simulink model "model_dyskretny"  (R2023a)
settings: Solver=VariableStepAuto  StartTime=0.0  StopTime=200  RelTol=1e-3
values from neighbouring files (symbols this model uses):
  a0 = 0.000531632    [zad1.m]    (also in zad2_8.m; zadanie_dodatkowe.m)
  a1 = 0.0207337    [zad1.m]    (also in zad2_8.m; zadanie_dodatkowe.m)
  a2 = 0.254652    [zad1.m]    (also in zad2_8.m; zadanie_dodatkowe.m)
  alpha1 = -0.3    [zad1.m]    (also in zad2_8.m; zadanie_dodatkowe.m)
  alpha2 = -0.55    [zad1.m]    (also in zad2_8.m; zadanie_dodatkowe.m)
  alpha3 = 0.4    [zad1.m]    (also in zad2_8.m; zadanie_dodatkowe.m)
  alpha4 = 0.21    [zad1.m]    (also in zad2_8.m; zadanie_dodatkowe.m)
  b0 = 0.00122807    [zad1.m]    (also in zad2_8.m; zadanie_dodatkowe.m)
  T = 5    [zad2_8.m]
undefined symbols (not defined in the file or in its folder): DiscIntNeverNeededParam
settings Model: Creator=adams  LastModifiedBy=adams

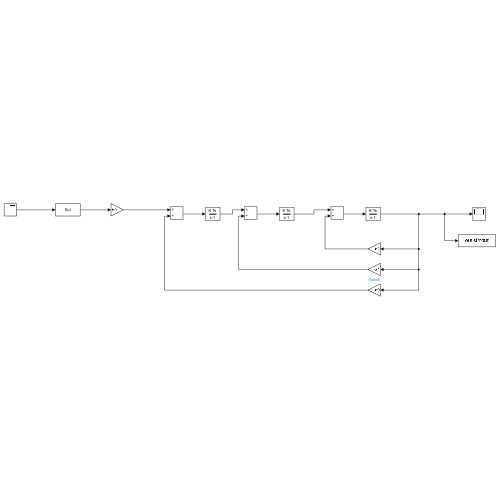
[thumbnail: Simulink's stored preview of the top-level diagram]
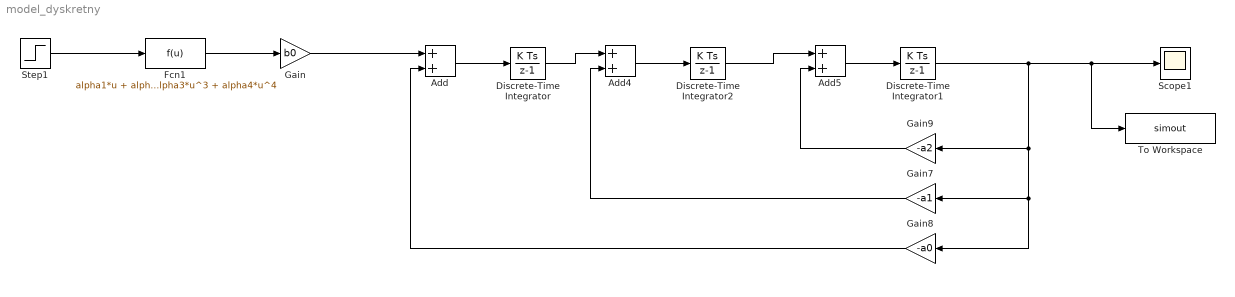
== system model_dyskretny ==
  Add : Sum
  Add4 : Sum
  Add5 : Sum
  Discrete-Time Integrator : DiscreteIntegrator  SampleTime=T  ICPrevOutput=DiscIntNeverNeededParam  ICPrevScaledInput=DiscIntNeverNeededParam
  Discrete-Time Integrator1 : DiscreteIntegrator  SampleTime=T  ICPrevOutput=DiscIntNeverNeededParam  ICPrevScaledInput=DiscIntNeverNeededParam
  Discrete-Time Integrator2 : DiscreteIntegrator  SampleTime=T  ICPrevOutput=DiscIntNeverNeededParam  ICPrevScaledInput=DiscIntNeverNeededParam
  Fcn1 : Fcn  Expr=alpha1*u + alpha2*u^2 + alpha3*u^3 + alpha4*u^4
  Gain : Gain  Gain=b0
  Gain7 : Gain  Gain=-a1
  Gain8 : Gain  Gain=-a0
  Gain9 : Gain  Gain=-a2
  Scope1 : Scope
  Step1 : Step  SampleTime=0
  To Workspace : ToWorkspace  VariableName=simout  SaveFormat=Structure With Time  SampleTime=-1
  wires:
  Gain/1 -> Add/1
  Step1/1 -> Fcn1/1
  Gain8/1 -> Add/2
  Gain7/1 -> Add4/2
  Discrete-Time Integrator/1 -> Add4/1
  Discrete-Time Integrator2/1 -> Add5/1
  Discrete-Time Integrator1/1 -> Gain7/1, Gain8/1, Gain9/1, To Workspace/1, Scope1/1
  Gain9/1 -> Add5/2
  Fcn1/1 -> Gain/1
  Add/1 -> Discrete-Time Integrator/1
  Add5/1 -> Discrete-Time Integrator1/1
  Add4/1 -> Discrete-Time Integrator2/1
